simulink model "Point2_IO_Linearization_HW2"  (R2024b)
settings: Solver=VariableStepAuto  StartTime=0.0  StopTime=15  RelTol=1e-3
InitFcn:
  | b_values = [b1, b2, b3];
  | assignin('base', 'b_values', b_values);
undefined symbols (not defined in the file): b1, b2, b3, current_b_index
libraries: robotmobilelib x1
settings Model: Creator=emanuela  LastModifiedBy=emanuela

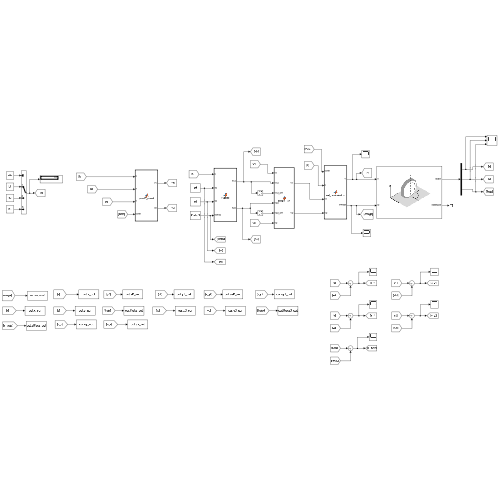
[thumbnail: Simulink's stored preview of the top-level diagram]
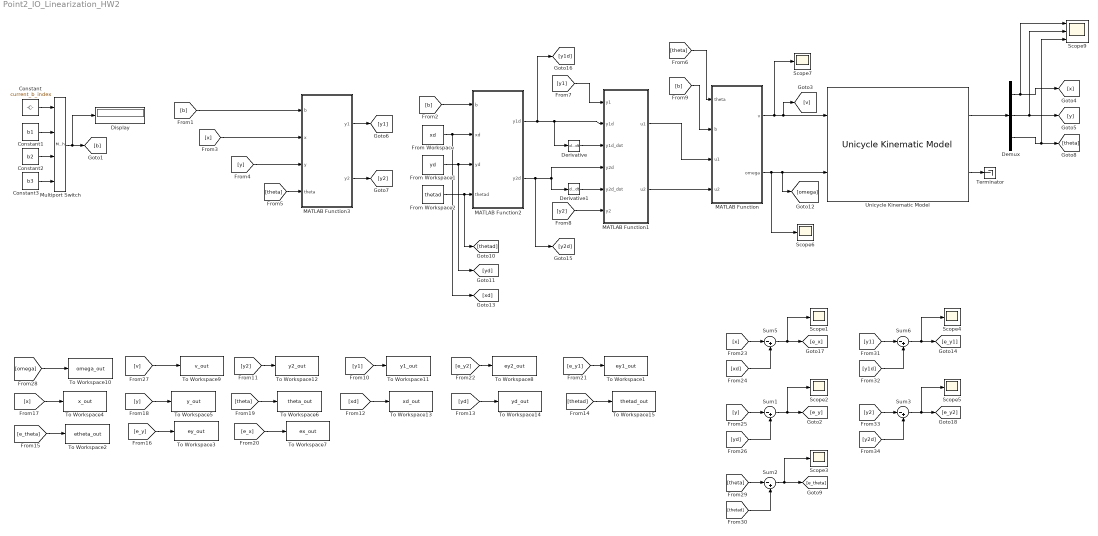
== system Point2_IO_Linearization_HW2 ==
  Constant : Constant  Value=current_b_index
  Constant1 : Constant  Value=b1
  Constant2 : Constant  Value=b2
  Constant3 : Constant  Value=b3
  Demux : Demux  Outputs=3
  Derivative : Derivative
  Derivative1 : Derivative
  Display : Display
  From Workspace : FromWorkspace  VariableName=xd
  From Workspace1 : FromWorkspace  VariableName=yd
  From Workspace2 : FromWorkspace  VariableName=thetad
  MATLAB Function : MATLAB Function  TreatAsAtomicUnit=on
  MATLAB Function1 : MATLAB Function  TreatAsAtomicUnit=on
  MATLAB Function2 : MATLAB Function  TreatAsAtomicUnit=on
  MATLAB Function3 : MATLAB Function  TreatAsAtomicUnit=on
  Multiport Switch : MultiPortSwitch  SaturateOnIntegerOverflow=off  InputSameDT=off
  Scope{1..7} (7 alike) : Scope
  Scope9 : Scope  NumInputPorts=3
  Sum{1..3,5..6} (5 alike) : Sum  Inputs=|-+
  Terminator : Terminator
  To Workspace1 : ToWorkspace  VariableName=ey1_out  SaveFormat=Structure With Time  SampleTime=-1
      settings: Save2DSignal=2-D array (concatenate along first dimension)
  To Workspace10 : ToWorkspace  VariableName=omega_out  SaveFormat=Structure With Time  SampleTime=-1
      settings: Save2DSignal=2-D array (concatenate along first dimension)
  To Workspace11 : ToWorkspace  VariableName=y1_out  SaveFormat=Structure With Time  SampleTime=-1
      settings: Save2DSignal=2-D array (concatenate along first dimension)
  To Workspace12 : ToWorkspace  VariableName=y2_out  SaveFormat=Structure With Time  SampleTime=-1
      settings: Save2DSignal=2-D array (concatenate along first dimension)
  To Workspace13 : ToWorkspace  VariableName=xd_out  SaveFormat=Structure With Time  SampleTime=-1
      settings: Save2DSignal=2-D array (concatenate along first dimension)
  To Workspace14 : ToWorkspace  VariableName=yd_out  SaveFormat=Structure With Time  SampleTime=-1
      settings: Save2DSignal=2-D array (concatenate along first dimension)
  To Workspace15 : ToWorkspace  VariableName=thetad_out  SaveFormat=Structure With Time  SampleTime=-1
      settings: Save2DSignal=2-D array (concatenate along first dimension)
  To Workspace2 : ToWorkspace  VariableName=etheta_out  SaveFormat=Structure With Time  SampleTime=-1
      settings: Save2DSignal=2-D array (concatenate along first dimension)
  To Workspace3 : ToWorkspace  VariableName=ey_out  SaveFormat=Structure With Time  SampleTime=-1
      settings: Save2DSignal=2-D array (concatenate along first dimension)
  To Workspace4 : ToWorkspace  VariableName=x_out  SaveFormat=Structure With Time  SampleTime=-1
      settings: Save2DSignal=2-D array (concatenate along first dimension)
  To Workspace5 : ToWorkspace  VariableName=y_out  SaveFormat=Structure With Time  SampleTime=-1
      settings: Save2DSignal=2-D array (concatenate along first dimension)
  To Workspace6 : ToWorkspace  VariableName=theta_out  SaveFormat=Structure With Time  SampleTime=-1
      settings: Save2DSignal=2-D array (concatenate along first dimension)
  To Workspace7 : ToWorkspace  VariableName=ex_out  SaveFormat=Structure With Time  SampleTime=-1
      settings: Save2DSignal=2-D array (concatenate along first dimension)
  To Workspace8 : ToWorkspace  VariableName=ey2_out  SaveFormat=Structure With Time  SampleTime=-1
      settings: Save2DSignal=2-D array (concatenate along first dimension)
  To Workspace9 : ToWorkspace  VariableName=v_out  SaveFormat=Structure With Time  SampleTime=-1
      settings: Save2DSignal=2-D array (concatenate along first dimension)
  Unicycle Kinematic Model : robotmobilelib/Unicycle Kinematic Model  VehicleInputs=Vehicle Speed & Heading Angular Velocity  WheelRadius=0.1  WheelSpeedRange=[-Inf Inf]  InitialState=[0; 0; 0]  SimulateUsing=Interpreted execution
  wires:
  Constant3/1 -> Multiport Switch/4
  Constant2/1 -> Multiport Switch/3
  Constant1/1 -> Multiport Switch/2
  [y] -> MATLAB Function3/3(y)
  MATLAB Function3/2(y2) -> [y2]
  MATLAB Function3/1(y1) -> [y1]
  [theta] -> MATLAB Function3/4(theta)
  Multiport Switch/1 -> Display/1, [b]
  [y1] -> MATLAB Function1/1(y1)
  MATLAB Function2/1(y1d) -> [y1d], Derivative/1, MATLAB Function1/2(y1d)
  [theta] -> MATLAB Function/1(theta)
  MATLAB Function1/1(u1) -> MATLAB Function/3(u1)
  MATLAB Function1/2(u2) -> MATLAB Function/4(u2)
  [b] -> MATLAB Function/2(b)
  Unicycle Kinematic Model/2 -> Terminator/1
  MATLAB Function/1(v) -> Scope7/1, [v], Unicycle Kinematic Model/1
  [x] -> MATLAB Function3/2(x)
  [b] -> MATLAB Function3/1(b)
  Demux/3 -> Scope9/3, [theta]
  Demux/2 -> Scope9/2, [y]
  Unicycle Kinematic Model/1 -> Demux/1
  From Workspace1/1 -> MATLAB Function2/3(yd), [yd]
  From Workspace/1 -> [xd], MATLAB Function2/2(xd)
  [b] -> MATLAB Function2/1(b)
  From Workspace2/1 -> [thetad], MATLAB Function2/4(thetad)
  [omega] -> To Workspace10/1
  MATLAB Function2/2(y2d) -> [y2d], MATLAB Function1/4(y2d), Derivative1/1
  [y2] -> MATLAB Function1/6(y2)
  [v] -> To Workspace9/1
  Derivative/1 -> MATLAB Function1/3(y1d_dot)
  Derivative1/1 -> MATLAB Function1/5(y2d_dot)
  [e_theta] -> To Workspace2/1
  [x] -> To Workspace4/1
  [theta] -> To Workspace6/1
  [y] -> To Workspace5/1
  [e_y] -> To Workspace3/1
  [e_x] -> To Workspace7/1
  [e_y1] -> To Workspace1/1
  [e_y2] -> To Workspace8/1
  [y1] -> To Workspace11/1
  [y2] -> To Workspace12/1
  Constant/1 -> Multiport Switch/1
  [xd] -> To Workspace13/1
  [yd] -> To Workspace14/1
  [thetad] -> To Workspace15/1
  [xd] -> Sum5/2
  [x] -> Sum5/1
  Sum5/1 -> Scope1/1, [e_x]
  Sum1/1 -> Scope2/1, [e_y]
  [y] -> Sum1/1
  [yd] -> Sum1/2
  [thetad] -> Sum2/2
  [theta] -> Sum2/1
  Sum2/1 -> [e_theta], Scope3/1
  [y1d] -> Sum6/2
  [y1] -> Sum6/1
  Sum6/1 -> Scope4/1, [e_y1]
  [y2d] -> Sum3/2
  Sum3/1 -> Scope5/1, [e_y2]
  [y2] -> Sum3/1
  Demux/1 -> Scope9/1, [x]
  MATLAB Function/2(omega) -> Scope6/1, Unicycle Kinematic Model/2, [omega]

== matlab function Point2_IO_Linearization_HW2/MATLAB Function ==
  data: v output; omega output; theta input; b input; u1 input; u2 input
function [v,omega] = vel_computation(theta,b,u1,u2)

T_theta=[cos(theta) -b*sin(theta); sin(theta) b*cos(theta)];

Tinv = inv(T_theta);

v = Tinv(1,:)*[u1; u2];
omega = Tinv(2,:)*[u1; u2];

end

== matlab function Point2_IO_Linearization_HW2/MATLAB Function2 ==
  data: b input; xd input; y1d output; yd input; thetad input; y2d output
function [y1d,y2d]  = outputs(b,xd,yd,thetad)

y1d=xd+b*cos(thetad);
y2d=yd+b*sin(thetad);

end

== matlab function Point2_IO_Linearization_HW2/MATLAB Function1 ==
  data: y1 input; y1d input; y1d_dot input; y2d input; y2d_dot input; y2 input; u1 output; u2 output
function [u1, u2] = linear_controller(y1, y1d, y1d_dot, y2d, y2d_dot,y2)
    
    k1 = 5;
    k2 = 5;

    % Control law (input-output linearization)
    u1 = y1d_dot + k1 * (y1d - y1);
    u2 = y2d_dot + k2 * (y2d - y2);
end

== matlab function Point2_IO_Linearization_HW2/MATLAB Function3 ==
  data: b input; x input; y1 output; y input; theta input; y2 output
function [y1,y2]  = pointB_coord(b,x,y,theta)

y1=x+b*cos(theta);
y2=y+b*sin(theta);

end
